simulink model "linear_regression1"  (Simulink 8.1)
settings: Solver=ode3  StartTime=0.0  StopTime=50  FixedStep=0.01  RelTol=1e-3
settings Model: Creator=root  LastModifiedBy=root
settings DataIOCC: SignalLoggingSaveFormat=Dataset
settings OptimizationCC: ExpressionDepthLimit=128
settings DebuggingCC: FcnCallInpInsideContextMsg=EnableAllAsError
settings GRTTargetCC: CombineOutputUpdateFcns=on  GRTInterface=off

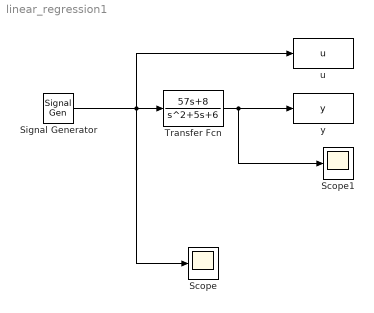
== system linear_regression1 ==
  Scope : Scope
  Scope1 : Scope
  Signal Generator : SignalGenerator  WaveForm=sawtooth  Frequency=0.1
  Transfer Fcn : TransferFcn  Numerator=[57 8 ]  Denominator=[1 5 6]
  u : ToWorkspace  VariableName=u  SampleTime=-1
  y : ToWorkspace  VariableName=y  SampleTime=-1
  wires:
  Signal Generator/1 -> Scope/1, Transfer Fcn/1, u/1
  Transfer Fcn/1 -> Scope1/1, y/1
